simulink model "PV_MPPT_SolarCharge_Control"  (R2021a)
settings: Solver=ode23tb  StartTime=0.0  StopTime=2  FixedStep=1  RelTol=1e-3
InitFcn:
  | %Fsw =1000 % PWM switching frequency
  | %dD = 1e-6;  MPPT Duty cycle
  | %BattCV = 55.4; Battery charging constant
undefined symbols (not defined in the file): Ion, Lithium
libraries: spsSeriesRLCBranchLib x3, simulink x2, spsDiodeLib x2, spsBatteryLib x1, spsMeanLib x1, spsMosfetLib x1, spsPVArrayLib x1, eePwmGenerator x1, spspowerguiLib x1
settings Model: Creator=Rodney Tan  LastModifiedBy=Jongo
settings SolverCC: AlgebraicLoopSolver=LineSearch
settings DataIOCC: ReturnWorkspaceOutputs=off
settings OptimizationCC: LifeSpan=inf
settings DebuggingCC: SFUnexpectedBacktrackingDiag=warning  SFNoUnconditionalDefaultTransitionDiag=warning  SFExecutionAtInitializationDiag=none  SFMachineParentedDataDiag=warning  ArithmeticOperatorsInVariantConditions=warning
settings SFSimCC: SimUseLocalCustomCode=off  CustomCodeUndefinedFunction=UseInterfaceOnly
settings RTWCC: RTWUseLocalCustomCode=off
settings CodeAppCC: StateflowObjectComments=on
settings GRTTargetCC: TargetLangStandard=C89/C90 (ANSI)
settings ConfigComp: CovMetricSettings=dw  CovSaveCumulativeToWorkspaceVar=on  CovSaveSingleToWorkspaceVar=on  CovExternalEMLEnable=off
settings SimscapeCC: SimscapeNormalizeSystem=off

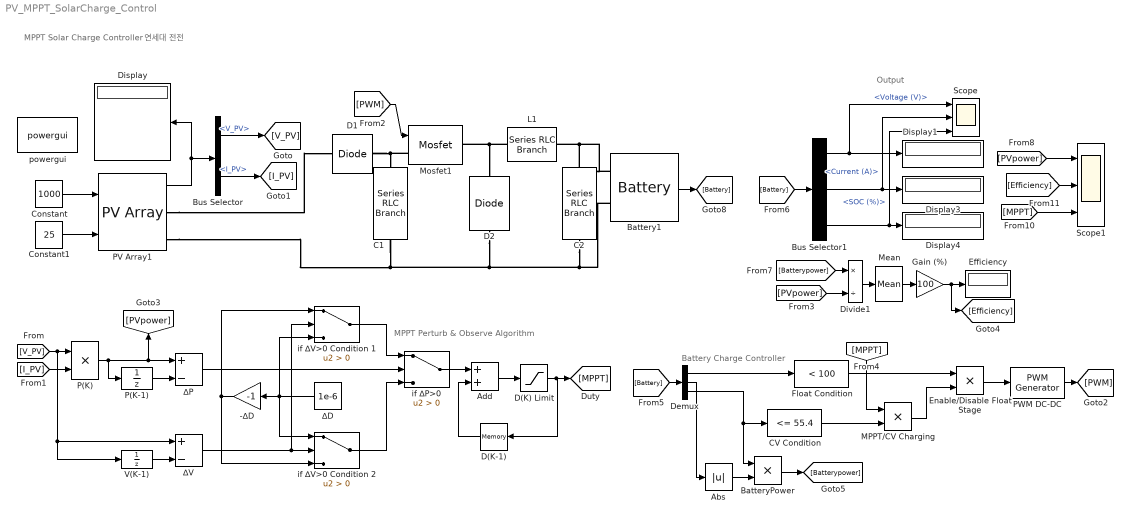
== system PV_MPPT_SolarCharge_Control ==
  note: Output
  note: MPPT Solar Charge Controller
      |  연세대 전전
  note: Battery Charge Controller
  note: MPPT Perturb & Observe Algorithm
  " C2" : spsSeriesRLCBranchLib/Series RLC Branch  LConnTagsString=__new0  RConnTagsString=__new0  BranchType=C  Resistance=0.1  Inductance=1e-3  SetiL0=off  InitialCurrent=0  Capacitance=1000e-6  Setx0=off  InitialVoltage=0  Measurements=None
  -∆D : Gain  Gain=-1
  Abs : Abs
  Add : Sum
  Battery1 : spsBatteryLib/Battery  BatType=Lithium-Ion  ShowTempParam=off  ThermalPreset=no  ShowAgeParam=off  NomV=48  NomQ=200  SOC=50  Batt_Tr=30  PresetModel=on  MaxQ=200  MinV=36  FullV=55.8714  Dis_rate=86.9565  R=0.0024  Normal_OP=180.8696  expZone="[51.8585      9.82609]"  current=[6.5 13 32.5]  Units=Time  Tci=20  NomT=20  T2=-30  MaxQ2=4.8  FullV2=7.1  Normal_OP2=5.655  expZone2="[6.58           1]"  Rca=0.6  ti=2000  Dp=0  Neq0=0  Tsim=1e6  Ta1=25  Qeol=5.4*0.9  Reol=0.013333*1.2  Char_age=[2.3478, 3]  Dis_age=[2.3478, 10]  N1=1500  N2=10500  N3=1000  N4=1400  Ta2=45  N5=950
  BatteryPower : Product
  Bus Selector : BusSelector  OutputSignals=V_PV,I_PV
  Bus Selector1 : BusSelector  OutputSignals=Voltage (V),Current (A),SOC (%)
  C1 : spsSeriesRLCBranchLib/Series RLC Branch  LConnTagsString=__new0  RConnTagsString=__new0  BranchType=C  Resistance=0.1  Inductance=1e-3  SetiL0=off  InitialCurrent=0  Capacitance=1000e-6  Setx0=off  InitialVoltage=0  Measurements=None
  CV Condition : simulink/Logic and Bit Operations/Compare To Constant  relop=<=  const=55.4  OutDataTypeStr=boolean
  Constant : Constant  Value=1000
  Constant1 : Constant  Value=25
  D(K) Limit : Saturate  UpperLimit=0.6  LowerLimit=0.4
  D(K-1) : Memory  InitialCondition=0.5  InheritSampleTime=on  LinearizeMemory=on  LinearizeAsDelay=on
  D1 : spsDiodeLib/Diode  Ron=0.001  Lon=0  Vf=0.8  IC=0  UseSnubber=0  Rs=inf  Cs=0  Measurements=off
  D2 : spsDiodeLib/Diode  Ron=0.001  Lon=0  Vf=0.5  IC=0  UseSnubber=0  Rs=inf  Cs=0  Measurements=off
  Demux : Demux  Outputs=3
  Display{,1,3..4} (4 alike) : Display
  Divide1 : Product  Inputs=*/
  Efficiency : Display
  Enable/Disable Float Stage : Product
  Float Condition : simulink/Logic and Bit Operations/Compare To Constant  relop=<  const=100  OutDataTypeStr=boolean
  Gain (%) : Gain  Gain=100
  L1 : spsSeriesRLCBranchLib/Series RLC Branch  LConnTagsString=__new0  RConnTagsString=__new0  BranchType=L  Resistance=1  Inductance=10e-3  SetiL0=off  InitialCurrent=0  Capacitance=1e-6  Setx0=off  InitialVoltage=0  Measurements=None
  MPPT/CV Charging : Product
  Mean : spsMeanLib/Mean  Freq=1  Vinit=0  Ts=0
  Mosfet1 : spsMosfetLib/Mosfet  Ron=0.02  Lon=0  Rd=0.01  Vfd=0  IC=0  Rs=1e5  Cs=inf  Measurements=off
  P(K) : Product
  P(K-1) : UnitDelay  SampleTime=-1  HasFrameUpgradeWarning=on
  PV Array1 : spsPVArrayLib/PV Array  Npar=2  Nser=4  PlotType=array @ 1000 W/m2 & specified temperatures  S_vec="[ 1000  500  100 ]"  Temp_C_vec="[ 45 25  ]"  ModuleName=User-defined  PlotWhenSelected=off  Pm=213.15  Ncell=60  Voc=36.3  Isc=7.84  Vm=29  Im=7.35  beta_Voc_pc=-0.36099  alpha_Isc_pc=0.102  beta_Voc=-0.13104  alpha_Isc=0.0079968  IL=7.8654  I0=2.9273e-10  nI=0.98119  Rsh=313.0553  Rs=0.39381  RobustModel=off  RobustCellTemperature=313.3991  BAL=off  Tc=1e-6  Tfilter=1e-5
  PWM DC-DC : eePwmGenerator/PWM Generator  CarrCount=Up  Tper=1/1000  Ts=0
  Scope : Scope  NumInputPorts=3
  Scope1 : Scope  NumInputPorts=3
  V(K-1) : UnitDelay  SampleTime=-1  HasFrameUpgradeWarning=on
  if ∆P>0 : Switch  Criteria=u2 > Threshold
  if ∆V>0 Condition 1 : Switch  Criteria=u2 > Threshold
  if ∆V>0 Condition 2 : Switch  Criteria=u2 > Threshold
  powergui : spspowerguiLib/powergui  Priority=1  SimulationMode=Discrete  SampleTime=1/1e5  frequency=60  Iterations=50  frequencyindice=0  Pbase=100e6  ErrMax=1e-4  UnitsV=kV  UnitsW=MW  buscounter=0  FunctionMessages=off  echomessages=off  EnableUseOfTLC=off  CurrentSourceSwitches=off  DisableSnubberDevices=off  DisableRonSwitches=off  DisableVfSwitches=off  DisplayEquations=off  AutomaticDiscreteSolvers=off  SolverType=Tustin/Backward Euler (TBE)  Interpol=off  ExternalGateDelay=off  methode=off  Ts=100  x0status=blocks  SPID=off  SwTol=0  HookPort=off  NonlinearTolerance=1e-4  nMaxIteration=100  ContinueOnMaxIteration=off  RestoreLinks=warning  ResistiveCurrentMeasurement=off  Frange=[0:2:500]  Ylog=off  Xlog=on  ShowGrid=off  save=off  variable=ZData  structure=0  ZoomFFT=off  StartTime=0.0  cycles=1  DisplayStyle=1  fundamental=60  FreqAxis=off  MaxFrequency=1000  frequencyindicesteady=1  RmsSteady=1  display=off
  ∆D : Constant  Value=1e-6
  ∆P : Sum  Inputs=+-
  ∆V : Sum  Inputs=+-
  wires:
  Battery1/1 -> [Battery]
  Constant/1 -> PV Array1/1
  Constant1/1 -> PV Array1/2
  PV Array1/1 -> Display/1, Bus Selector/1
  Bus Selector/1 -> [V_PV]  "<V_PV>"
  Bus Selector/2 -> [I_PV]  "<I_PV>"
  D(K) Limit/1 -> D(K-1)/1, [MPPT]
  CV Condition/1 -> MPPT/CV Charging/2
  Demux/3 -> CV Condition/1, BatteryPower/1
  [V_PV] -> V(K-1)/1, ∆V/1, P(K)/1
  Gain (%)/1 -> [Efficiency], Efficiency/1
  PWM DC-DC/1 -> [PWM]
  ∆D/1 -> if ∆V>0 Condition 2/1, -∆D/1, if ∆V>0 Condition 1/3
  P(K-1)/1 -> ∆P/2
  if ∆V>0 Condition 2/1 -> if ∆P>0/3
  ∆V/1 -> if ∆V>0 Condition 2/2, if ∆V>0 Condition 1/2
  -∆D/1 -> if ∆V>0 Condition 2/3, if ∆V>0 Condition 1/1
  ∆P/1 -> if ∆P>0/2
  Add/1 -> D(K) Limit/1
  Demux/1 -> Float Condition/1
  if ∆P>0/1 -> Add/1
  Float Condition/1 -> Enable/Disable Float Stage/1
  D(K-1)/1 -> Add/2
  Divide1/1 -> Mean/1
  [Battery] -> Demux/1
  MPPT/CV Charging/1 -> Enable/Disable Float Stage/2
  V(K-1)/1 -> ∆V/2
  Enable/Disable Float Stage/1 -> PWM DC-DC/1
  Abs/1 -> BatteryPower/2
  P(K)/1 -> P(K-1)/1, ∆P/1, [PVpower]
  Mean/1 -> Gain (%)/1
  Demux/2 -> Abs/1
  if ∆V>0 Condition 1/1 -> if ∆P>0/1
  [I_PV] -> P(K)/2
  [PVpower] -> Divide1/2
  [MPPT] -> MPPT/CV Charging/1
  [PWM] -> Mosfet1/1
  Bus Selector1/1 -> Display1/1, Scope/1  "<Voltage (V)>"
  Bus Selector1/2 -> Display3/1, Scope/2  "<Current (A)>"
  Bus Selector1/3 -> Scope/3, Display4/1  "<SOC (%)>"
  [Battery] -> Bus Selector1/1
  [Batterypower] -> Divide1/1
  BatteryPower/1 -> [Batterypower]
  [PVpower] -> Scope1/1
  [Efficiency] -> Scope1/2
  [MPPT] -> Scope1/3
  connections:
  " C2"/LConn1 -- Battery1/LConn1 -- L1/RConn1
  D1/RConn1 -- Mosfet1/LConn1 -- C1/LConn1
  " C2"/RConn1 -- Battery1/LConn2 -- D2/LConn1 -- PV Array1/RConn2 -- C1/RConn1
  L1/LConn1 -- Mosfet1/RConn1 -- D2/RConn1
  PV Array1/RConn1 -- D1/LConn1
